simulink model "case8"  (R2024b)
settings: Solver=FixedStepAuto  StartTime=0  StopTime=1  FixedStep=1e-7  RelTol=1e-3
values from neighbouring files (symbols this model uses):
  SG_D_1_D = 0.01056    [IEEE9_case_parameters.m]    (also in case1_parameters.m; case2_parameters.m; case3_parameters.m; case4_parameters.m)
  SG_D_1_EnableSaturation = 0    [IEEE9_case_parameters.m]    (also in case1_parameters.m; case2_parameters.m; case3_parameters.m; case4_parameters.m)
  SG_D_1_f0 = 60    [IEEE9_case_parameters.m]    (also in case1_parameters.m; case2_parameters.m; case3_parameters.m; case4_parameters.m)
  SG_D_1_H = 7.5    [IEEE9_case_parameters.m]    (also in case1_parameters.m; case2_parameters.m; case3_parameters.m; case4_parameters.m)
  SG_D_1_K_A = 20    [IEEE9_case_parameters.m]    (also in case1_parameters.m; case2_parameters.m; case3_parameters.m; case4_parameters.m)
  SG_D_1_K_E = 1.000000e+1    (= 10)    [IEEE9_case_parameters.m]    (also in case1_parameters.m; case2_parameters.m; case3_parameters.m; case4_parameters.m)
  SG_D_1_K_F = 2.363    [IEEE9_case_parameters.m]    (also in case1_parameters.m; case2_parameters.m; case3_parameters.m; case4_parameters.m)
  SG_D_1_K_s = 0.5    [IEEE9_case_parameters.m]    (also in case1_parameters.m = 5; case2_parameters.m = 5; case3_parameters.m = 5; case4_parameters.m = 5)
  SG_D_1_R_a = 0.001088    [IEEE9_case_parameters.m]    (also in case1_parameters.m; case2_parameters.m; case3_parameters.m; case4_parameters.m)
  SG_D_1_S_A = 1    [IEEE9_case_parameters.m]    (also in case1_parameters.m; case2_parameters.m; case3_parameters.m; case4_parameters.m)
  SG_D_1_S_B = 0.103    [IEEE9_case_parameters.m]    (also in case1_parameters.m; case2_parameters.m; case3_parameters.m; case4_parameters.m)
  SG_D_1_S_N = 10.659857    [IEEE9_case_parameters.m]    (also in case1_parameters.m; case2_parameters.m; case3_parameters.m; case4_parameters.m)
  SG_D_1_SpeedPara = 200    [IEEE9_case_parameters.m]    (also in case1_parameters.m; case2_parameters.m; case3_parameters.m; case4_parameters.m)
  SG_D_1_T_0 = 0.720173    [IEEE9_case_parameters.m]    (also in case1_parameters.m = 0.755522; case2_parameters.m = 0.808931; case3_parameters.m = 0.869402; case4_parameters.m = 0.729316)
  SG_D_1_T_1 = 0.3    [IEEE9_case_parameters.m]    (also in case1_parameters.m; case2_parameters.m; case3_parameters.m; case4_parameters.m)
  SG_D_1_T_2 = 0.05    [IEEE9_case_parameters.m]    (also in case1_parameters.m; case2_parameters.m; case3_parameters.m; case4_parameters.m)
  SG_D_1_T_3 = 0.02    [IEEE9_case_parameters.m]    (also in case1_parameters.m; case2_parameters.m; case3_parameters.m; case4_parameters.m)
  SG_D_1_T_4 = 0.005    [IEEE9_case_parameters.m]    (also in case1_parameters.m; case2_parameters.m; case3_parameters.m; case4_parameters.m)
  SG_D_1_T_A = 0.02    [IEEE9_case_parameters.m]    (also in case1_parameters.m; case2_parameters.m; case3_parameters.m; case4_parameters.m)
  SG_D_1_T_dd = 8.000000e+0    (= 8)    [IEEE9_case_parameters.m]    (also in case1_parameters.m; case2_parameters.m; case3_parameters.m; case4_parameters.m)
  SG_D_1_T_ddd = 0.04    [IEEE9_case_parameters.m]    (also in case1_parameters.m; case2_parameters.m; case3_parameters.m; case4_parameters.m)
  SG_D_1_T_E = 0.314    [IEEE9_case_parameters.m]    (also in case1_parameters.m; case2_parameters.m; case3_parameters.m; case4_parameters.m)
  SG_D_1_T_F = 0.35    [IEEE9_case_parameters.m]    (also in case1_parameters.m; case2_parameters.m; case3_parameters.m; case4_parameters.m)
  SG_D_1_T_qd = 0.8    [IEEE9_case_parameters.m]    (also in case1_parameters.m; case2_parameters.m; case3_parameters.m; case4_parameters.m)
  SG_D_1_T_qdd = 0.02    [IEEE9_case_parameters.m]    (also in case1_parameters.m; case2_parameters.m; case3_parameters.m; case4_parameters.m)
  SG_D_1_T_speed = 0.1    [IEEE9_case_parameters.m]    (also in case1_parameters.m = 200; case2_parameters.m = 200; case3_parameters.m = 200; case4_parameters.m = 200)
  SG_D_1_T_w = 0.5    [IEEE9_case_parameters.m]    (also in case1_parameters.m; case2_parameters.m; case3_parameters.m; case4_parameters.m)
  SG_D_1_V_ref = 1.990276    [IEEE9_case_parameters.m]    (also in case1_parameters.m = 2.042296; case2_parameters.m = 2.051388; case3_parameters.m = 2.089584; case4_parameters.m = 2.01845)
  SG_D_1_w_ref = 376.991118    [IEEE9_case_parameters.m]    (also in case1_parameters.m; case2_parameters.m; case3_parameters.m; case4_parameters.m)
  SG_D_1_wb = 6.000000e+1    (= 60)    [IEEE9_case_parameters.m]    (also in case1_parameters.m; case2_parameters.m; case3_parameters.m; case4_parameters.m)
  SG_D_1_x_d = 1.9    [IEEE9_case_parameters.m]    (also in case1_parameters.m; case2_parameters.m; case3_parameters.m; case4_parameters.m)
  SG_D_1_x_dd = 0.302    [IEEE9_case_parameters.m]    (also in case1_parameters.m; case2_parameters.m; case3_parameters.m; case4_parameters.m)
  SG_D_1_x_ddd = 0.204    [IEEE9_case_parameters.m]    (also in case1_parameters.m; case2_parameters.m; case3_parameters.m; case4_parameters.m)
  SG_D_1_x_l = 0.05    [IEEE9_case_parameters.m]    (also in case1_parameters.m; case2_parameters.m; case3_parameters.m; case4_parameters.m)
  SG_D_1_x_q = 1.3    [IEEE9_case_parameters.m]    (also in case1_parameters.m; case2_parameters.m; case3_parameters.m; case4_parameters.m)
  SG_D_1_x_qd = 0.5    [IEEE9_case_parameters.m]    (also in case1_parameters.m; case2_parameters.m; case3_parameters.m; case4_parameters.m)
  SG_D_1_x_qdd = 0.3    [IEEE9_case_parameters.m]    (also in case1_parameters.m; case2_parameters.m; case3_parameters.m; case4_parameters.m)
  SG_D_2_D = 0.02    [IEEE9_case_parameters.m]    (also in case1_parameters.m; case2_parameters.m; case3_parameters.m; case4_parameters.m)
  SG_D_2_EnableSaturation = 0    [IEEE9_case_parameters.m]    (also in case1_parameters.m; case2_parameters.m; case3_parameters.m; case4_parameters.m)
  SG_D_2_f0 = 60    [IEEE9_case_parameters.m]    (also in case1_parameters.m; case2_parameters.m; case3_parameters.m; case4_parameters.m)
  SG_D_2_H = 8.000000e+0    (= 8)    [IEEE9_case_parameters.m]    (also in case1_parameters.m; case2_parameters.m; case3_parameters.m; case4_parameters.m)
  SG_D_2_K_A = 20    [IEEE9_case_parameters.m]    (also in case1_parameters.m; case2_parameters.m; case3_parameters.m; case4_parameters.m)
  SG_D_2_K_E = 1.000000e+1    (= 10)    [IEEE9_case_parameters.m]    (also in case1_parameters.m; case2_parameters.m; case3_parameters.m; case4_parameters.m)
  SG_D_2_K_F = 2.363    [IEEE9_case_parameters.m]    (also in case1_parameters.m; case2_parameters.m; case3_parameters.m; case4_parameters.m)
  SG_D_2_K_s = 0.5    [IEEE9_case_parameters.m]    (also in case1_parameters.m = 4; case2_parameters.m = 4; case3_parameters.m = 4; case4_parameters.m = 4)
  SG_D_2_R_a = 0.001088    [IEEE9_case_parameters.m]    (also in case1_parameters.m; case2_parameters.m; case3_parameters.m; case4_parameters.m)
  SG_D_2_S_A = 1    [IEEE9_case_parameters.m]    (also in case1_parameters.m; case2_parameters.m; case3_parameters.m; case4_parameters.m)
  SG_D_2_S_B = 0.103    [IEEE9_case_parameters.m]    (also in case1_parameters.m; case2_parameters.m; case3_parameters.m; case4_parameters.m)
  SG_D_2_S_N = 10.659857    [IEEE9_case_parameters.m]    (also in case1_parameters.m; case2_parameters.m; case3_parameters.m; case4_parameters.m)
  SG_D_2_SpeedPara = 200    [IEEE9_case_parameters.m]    (also in case1_parameters.m; case2_parameters.m; case3_parameters.m; case4_parameters.m)
  SG_D_2_T_0 = 1.632913    [IEEE9_case_parameters.m]    (also in case1_parameters.m = 1.632925; case2_parameters.m = 1.632915; case3_parameters.m = 1.632914; case4_parameters.m = 1.632927)
  SG_D_2_T_1 = 0.2    [IEEE9_case_parameters.m]    (also in case1_parameters.m; case2_parameters.m; case3_parameters.m; case4_parameters.m)
  SG_D_2_T_2 = 0.05    [IEEE9_case_parameters.m]    (also in case1_parameters.m; case2_parameters.m; case3_parameters.m; case4_parameters.m)
  SG_D_2_T_3 = 0.02    [IEEE9_case_parameters.m]    (also in case1_parameters.m; case2_parameters.m; case3_parameters.m; case4_parameters.m)
  SG_D_2_T_4 = 0.005    [IEEE9_case_parameters.m]    (also in case1_parameters.m; case2_parameters.m; case3_parameters.m; case4_parameters.m)
  SG_D_2_T_A = 0.02    [IEEE9_case_parameters.m]    (also in case1_parameters.m; case2_parameters.m; case3_parameters.m; case4_parameters.m)
  SG_D_2_T_dd = 7.9    [IEEE9_case_parameters.m]    (also in case1_parameters.m; case2_parameters.m; case3_parameters.m; case4_parameters.m)
  SG_D_2_T_ddd = 0.04    [IEEE9_case_parameters.m]    (also in case1_parameters.m; case2_parameters.m; case3_parameters.m; case4_parameters.m)
  SG_D_2_T_E = 0.314    [IEEE9_case_parameters.m]    (also in case1_parameters.m; case2_parameters.m; case3_parameters.m; case4_parameters.m)
  SG_D_2_T_F = 0.35    [IEEE9_case_parameters.m]    (also in case1_parameters.m; case2_parameters.m; case3_parameters.m; case4_parameters.m)
  SG_D_2_T_qd = 0.8    [IEEE9_case_parameters.m]    (also in case1_parameters.m; case2_parameters.m; case3_parameters.m; case4_parameters.m)
  SG_D_2_T_qdd = 0.015    [IEEE9_case_parameters.m]    (also in case1_parameters.m; case2_parameters.m; case3_parameters.m; case4_parameters.m)
  SG_D_2_T_speed = 0.1    [IEEE9_case_parameters.m]    (also in case1_parameters.m = 150; case2_parameters.m = 150; case3_parameters.m = 150; case4_parameters.m = 150)
  SG_D_2_T_w = 0.35    [IEEE9_case_parameters.m]    (also in case1_parameters.m; case2_parameters.m; case3_parameters.m; case4_parameters.m)
  SG_D_2_V_ref = 2.58547    [IEEE9_case_parameters.m]    (also in case1_parameters.m = 2.597896; case2_parameters.m = 2.587136; case3_parameters.m = 2.586042; case4_parameters.m = 2.599679)
  SG_D_2_w_ref = 376.991118    [IEEE9_case_parameters.m]    (also in case1_parameters.m; case2_parameters.m; case3_parameters.m; case4_parameters.m)
  SG_D_2_wb = 6.000000e+1    (= 60)    [IEEE9_case_parameters.m]    (also in case1_parameters.m; case2_parameters.m; case3_parameters.m; case4_parameters.m)
  SG_D_2_x_d = 1.8    [IEEE9_case_parameters.m]    (also in case1_parameters.m; case2_parameters.m; case3_parameters.m; case4_parameters.m)
  SG_D_2_x_dd = 0.302    [IEEE9_case_parameters.m]    (also in case1_parameters.m; case2_parameters.m; case3_parameters.m; case4_parameters.m)
  SG_D_2_x_ddd = 0.204    [IEEE9_case_parameters.m]    (also in case1_parameters.m; case2_parameters.m; case3_parameters.m; case4_parameters.m)
  SG_D_2_x_l = 0.05    [IEEE9_case_parameters.m]    (also in case1_parameters.m; case2_parameters.m; case3_parameters.m; case4_parameters.m)
  SG_D_2_x_q = 1.25    [IEEE9_case_parameters.m]    (also in case1_parameters.m; case2_parameters.m; case3_parameters.m; case4_parameters.m)
  SG_D_2_x_qd = 0.5    [IEEE9_case_parameters.m]    (also in case1_parameters.m; case2_parameters.m; case3_parameters.m; case4_parameters.m)
  SG_D_2_x_qdd = 0.3    [IEEE9_case_parameters.m]    (also in case1_parameters.m; case2_parameters.m; case3_parameters.m; case4_parameters.m)
  SG_D_3_D = 0.02    [IEEE9_case_parameters.m]    (also in case1_parameters.m; case2_parameters.m; case3_parameters.m; case4_parameters.m)
  SG_D_3_EnableSaturation = 0    [IEEE9_case_parameters.m]    (also in case1_parameters.m; case2_parameters.m; case3_parameters.m; case4_parameters.m)
  SG_D_3_f0 = 60    [IEEE9_case_parameters.m]    (also in case1_parameters.m; case2_parameters.m; case3_parameters.m; case4_parameters.m)
  SG_D_3_H = 7.7    [IEEE9_case_parameters.m]    (also in case1_parameters.m; case2_parameters.m; case3_parameters.m; case4_parameters.m)
  SG_D_3_K_A = 20    [IEEE9_case_parameters.m]    (also in case1_parameters.m; case2_parameters.m; case3_parameters.m; case4_parameters.m)
  SG_D_3_K_E = 1.000000e+1    (= 10)    [IEEE9_case_parameters.m]    (also in case1_parameters.m; case2_parameters.m; case3_parameters.m; case4_parameters.m)
  SG_D_3_K_F = 2.363    [IEEE9_case_parameters.m]    (also in case1_parameters.m; case2_parameters.m; case3_parameters.m; case4_parameters.m)
  SG_D_3_K_s = 0.2    [IEEE9_case_parameters.m]    (also in case1_parameters.m = 2; case2_parameters.m = 2; case3_parameters.m = 2; case4_parameters.m = 2)
  SG_D_3_R_a = 0.001088    [IEEE9_case_parameters.m]    (also in case1_parameters.m; case2_parameters.m; case3_parameters.m; case4_parameters.m)
  SG_D_3_S_A = 1    [IEEE9_case_parameters.m]    (also in case1_parameters.m; case2_parameters.m; case3_parameters.m; case4_parameters.m)
  SG_D_3_S_B = 0.103    [IEEE9_case_parameters.m]    (also in case1_parameters.m; case2_parameters.m; case3_parameters.m; case4_parameters.m)
  SG_D_3_S_N = 10.659857    [IEEE9_case_parameters.m]    (also in case1_parameters.m; case2_parameters.m; case3_parameters.m; case4_parameters.m)
  SG_D_3_SpeedPara = 200    [IEEE9_case_parameters.m]    (also in case1_parameters.m; case2_parameters.m; case3_parameters.m; case4_parameters.m)
  SG_D_3_T_0 = 0.850788    [IEEE9_case_parameters.m]    (also in case1_parameters.m = 0.850786; case2_parameters.m = 0.850787; case3_parameters.m; case4_parameters.m = 0.850786)
  SG_D_3_T_1 = 0.2    [IEEE9_case_parameters.m]    (also in case1_parameters.m; case2_parameters.m; case3_parameters.m; case4_parameters.m)
  SG_D_3_T_2 = 0.05    [IEEE9_case_parameters.m]    (also in case1_parameters.m; case2_parameters.m; case3_parameters.m; case4_parameters.m)
  SG_D_3_T_3 = 0.02    [IEEE9_case_parameters.m]    (also in case1_parameters.m; case2_parameters.m; case3_parameters.m; case4_parameters.m)
  SG_D_3_T_4 = 0.005    [IEEE9_case_parameters.m]    (also in case1_parameters.m; case2_parameters.m; case3_parameters.m; case4_parameters.m)
  SG_D_3_T_A = 0.02    [IEEE9_case_parameters.m]    (also in case1_parameters.m; case2_parameters.m; case3_parameters.m; case4_parameters.m)
  SG_D_3_T_dd = 8.1    [IEEE9_case_parameters.m]    (also in case1_parameters.m; case2_parameters.m; case3_parameters.m; case4_parameters.m)
  SG_D_3_T_ddd = 0.04    [IEEE9_case_parameters.m]    (also in case1_parameters.m; case2_parameters.m; case3_parameters.m; case4_parameters.m)
  SG_D_3_T_E = 0.314    [IEEE9_case_parameters.m]    (also in case1_parameters.m; case2_parameters.m; case3_parameters.m; case4_parameters.m)
  SG_D_3_T_F = 0.35    [IEEE9_case_parameters.m]    (also in case1_parameters.m; case2_parameters.m; case3_parameters.m; case4_parameters.m)
  SG_D_3_T_qd = 0.8    [IEEE9_case_parameters.m]    (also in case1_parameters.m; case2_parameters.m; case3_parameters.m; case4_parameters.m)
  SG_D_3_T_qdd = 0.015    [IEEE9_case_parameters.m]    (also in case1_parameters.m; case2_parameters.m; case3_parameters.m; case4_parameters.m)
  SG_D_3_T_speed = 0.1    [IEEE9_case_parameters.m]    (also in case1_parameters.m = 180; case2_parameters.m = 180; case3_parameters.m = 180; case4_parameters.m = 180)
  SG_D_3_T_w = 0.4    [IEEE9_case_parameters.m]    (also in case1_parameters.m; case2_parameters.m; case3_parameters.m; case4_parameters.m)
  SG_D_3_V_ref = 1.892727    [IEEE9_case_parameters.m]    (also in case1_parameters.m = 1.906439; case2_parameters.m = 1.895535; case3_parameters.m = 1.892105; case4_parameters.m = 1.906598)
  SG_D_3_w_ref = 376.991118    [IEEE9_case_parameters.m]    (also in case1_parameters.m; case2_parameters.m; case3_parameters.m; case4_parameters.m)
  SG_D_3_wb = 6.000000e+1    (= 60)    [IEEE9_case_parameters.m]    (also in case1_parameters.m; case2_parameters.m; case3_parameters.m; case4_parameters.m)
  SG_D_3_x_d = 1.85    [IEEE9_case_parameters.m]    (also in case1_parameters.m; case2_parameters.m; case3_parameters.m; case4_parameters.m)
  SG_D_3_x_dd = 0.302    [IEEE9_case_parameters.m]    (also in case1_parameters.m; case2_parameters.m; case3_parameters.m; case4_parameters.m)
  SG_D_3_x_ddd = 0.204    [IEEE9_case_parameters.m]    (also in case1_parameters.m; case2_parameters.m; case3_parameters.m; case4_parameters.m)
  SG_D_3_x_l = 0.05    [IEEE9_case_parameters.m]    (also in case1_parameters.m; case2_parameters.m; case3_parameters.m; case4_parameters.m)
  SG_D_3_x_q = 1.2    [IEEE9_case_parameters.m]    (also in case1_parameters.m; case2_parameters.m; case3_parameters.m; case4_parameters.m)
  SG_D_3_x_qd = 0.5    [IEEE9_case_parameters.m]    (also in case1_parameters.m; case2_parameters.m; case3_parameters.m; case4_parameters.m)
  SG_D_3_x_qdd = 0.3    [IEEE9_case_parameters.m]    (also in case1_parameters.m; case2_parameters.m; case3_parameters.m; case4_parameters.m)
(part 1 of 12)
settings Model: Creator=Greg  LastModifiedBy=Greg

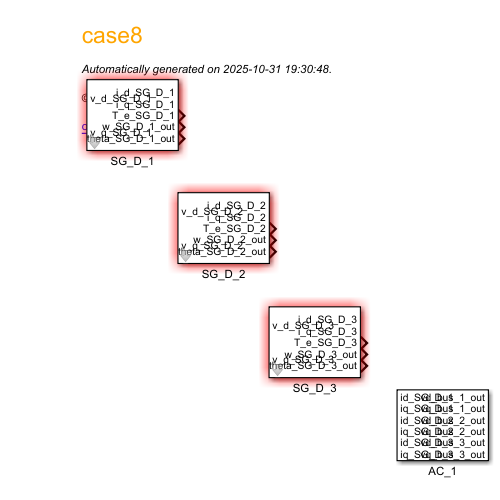
[thumbnail: Simulink's stored preview of the top-level diagram]
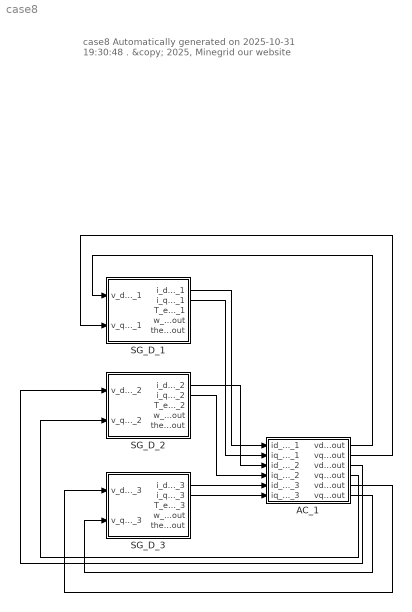
== system case8 ==
  note: case8
      | Automatically generated on 2025-10-31 19:30:48 .
      | &copy; 2025, Minegrid
      | our website
  AC_1 : Subsystem  mask(AC_1){}
      mask help: Parameters Interface of AC_1
  SG_D_1 : Subsystem  mask(SG_D_1){T_0=SG_D_1_T_0, w_ref=SG_D_1_w_ref, V_ref=SG_D_1_V_ref, x_d=SG_D_1_x_d, x_dd=SG_D_1_x_dd, x_ddd=SG_D_1_x_ddd, x_q=SG_D_1_x_q, x_qd=SG_D_1_x_qd, x_qdd=SG_D_1_x_qdd, x_l=SG_D_1_x_l, R_a=SG_D_1_R_a, T_dd=SG_D_1_T_dd, T_ddd=SG_D_1_T_ddd, T_qd=SG_D_1_T_qd, T_qdd=SG_D_1_T_qdd, H=SG_D_1_H, D=SG_D_1_D, SpeedPara=SG_D_1_SpeedPara, K_A=SG_D_1_K_A, EnableSaturation=SG_D_1_EnableSaturation, f0=SG_D_1_f0, T_speed=SG_D_1_T_speed, T_E=SG_D_1_T_E, T_A=SG_D_1_T_A, T_F=SG_D_1_T_F, K_E=SG_D_1_K_E, K_F=SG_D_1_K_F, K_s=SG_D_1_K_s, T_1=SG_D_1_T_1, T_2=SG_D_1_T_2, T_3=SG_D_1_T_3, T_4=SG_D_1_T_4, T_w=SG_D_1_T_w, wb=SG_D_1_wb, S_A=SG_D_1_S_A, S_B=SG_D_1_S_B, S_N=SG_D_1_S_N}
      mask help: Parameters Interface of SG_D_1
  SG_D_2 : Subsystem  mask(SG_D_2){T_0=SG_D_2_T_0, w_ref=SG_D_2_w_ref, V_ref=SG_D_2_V_ref, x_d=SG_D_2_x_d, x_dd=SG_D_2_x_dd, x_ddd=SG_D_2_x_ddd, x_q=SG_D_2_x_q, x_qd=SG_D_2_x_qd, x_qdd=SG_D_2_x_qdd, x_l=SG_D_2_x_l, R_a=SG_D_2_R_a, T_dd=SG_D_2_T_dd, T_ddd=SG_D_2_T_ddd, T_qd=SG_D_2_T_qd, T_qdd=SG_D_2_T_qdd, H=SG_D_2_H, D=SG_D_2_D, SpeedPara=SG_D_2_SpeedPara, K_A=SG_D_2_K_A, EnableSaturation=SG_D_2_EnableSaturation, f0=SG_D_2_f0, T_speed=SG_D_2_T_speed, T_E=SG_D_2_T_E, T_A=SG_D_2_T_A, T_F=SG_D_2_T_F, K_E=SG_D_2_K_E, K_F=SG_D_2_K_F, K_s=SG_D_2_K_s, T_1=SG_D_2_T_1, T_2=SG_D_2_T_2, T_3=SG_D_2_T_3, T_4=SG_D_2_T_4, T_w=SG_D_2_T_w, wb=SG_D_2_wb, S_A=SG_D_2_S_A, S_B=SG_D_2_S_B, S_N=SG_D_2_S_N}
      mask help: Parameters Interface of SG_D_2
  SG_D_3 : Subsystem  mask(SG_D_3){T_0=SG_D_3_T_0, w_ref=SG_D_3_w_ref, V_ref=SG_D_3_V_ref, x_d=SG_D_3_x_d, x_dd=SG_D_3_x_dd, x_ddd=SG_D_3_x_ddd, x_q=SG_D_3_x_q, x_qd=SG_D_3_x_qd, x_qdd=SG_D_3_x_qdd, x_l=SG_D_3_x_l, R_a=SG_D_3_R_a, T_dd=SG_D_3_T_dd, T_ddd=SG_D_3_T_ddd, T_qd=SG_D_3_T_qd, T_qdd=SG_D_3_T_qdd, H=SG_D_3_H, D=SG_D_3_D, SpeedPara=SG_D_3_SpeedPara, K_A=SG_D_3_K_A, EnableSaturation=SG_D_3_EnableSaturation, f0=SG_D_3_f0, T_speed=SG_D_3_T_speed, T_E=SG_D_3_T_E, T_A=SG_D_3_T_A, T_F=SG_D_3_T_F, K_E=SG_D_3_K_E, K_F=SG_D_3_K_F, K_s=SG_D_3_K_s, T_1=SG_D_3_T_1, T_2=SG_D_3_T_2, T_3=SG_D_3_T_3, T_4=SG_D_3_T_4, T_w=SG_D_3_T_w, wb=SG_D_3_wb, S_A=SG_D_3_S_A, S_B=SG_D_3_S_B, S_N=SG_D_3_S_N}
      mask help: Parameters Interface of SG_D_3
  wires:
  SG_D_2/2(i_q_SG_D_2) -> AC_1/4(iq_SG_D_2)
  SG_D_1/2(i_q_SG_D_1) -> AC_1/2(iq_SG_D_1)
  SG_D_1/1(i_d_SG_D_1) -> AC_1/1(id_SG_D_1)
  SG_D_2/1(i_d_SG_D_2) -> AC_1/3(id_SG_D_2)
  AC_1/1(vd_bus_1_out) -> SG_D_1/1(v_d_SG_D_1)
  SG_D_3/1(i_d_SG_D_3) -> AC_1/5(id_SG_D_3)
  AC_1/2(vq_bus_1_out) -> SG_D_1/2(v_q_SG_D_1)
  SG_D_3/2(i_q_SG_D_3) -> AC_1/6(iq_SG_D_3)
  AC_1/3(vd_bus_2_out) -> SG_D_2/1(v_d_SG_D_2)
  AC_1/4(vq_bus_2_out) -> SG_D_2/2(v_q_SG_D_2)
  AC_1/5(vd_bus_3_out) -> SG_D_3/1(v_d_SG_D_3)
  AC_1/6(vq_bus_3_out) -> SG_D_3/2(v_q_SG_D_3)

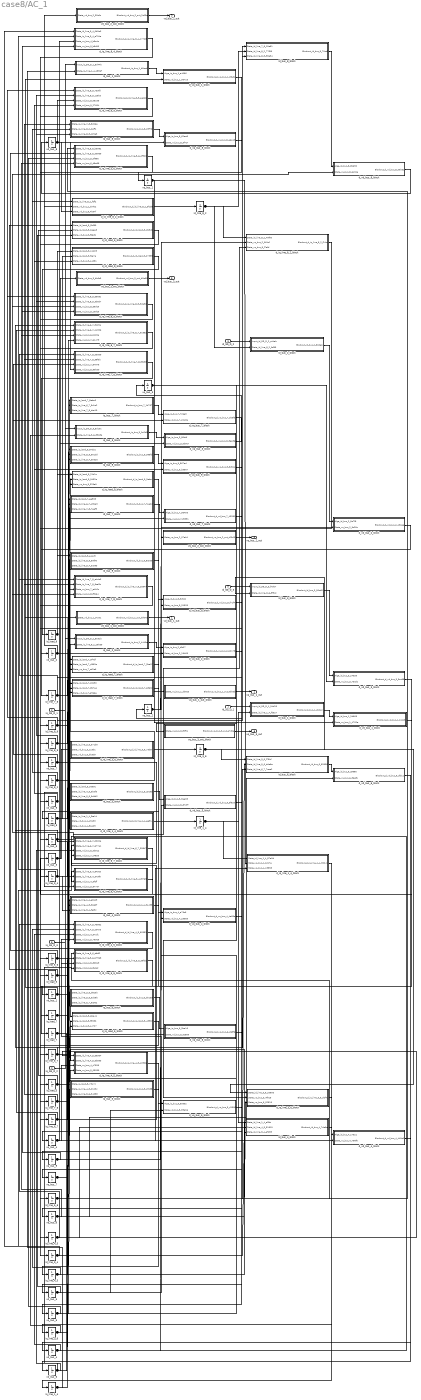
== system case8/AC_1 ==
  id_SG_D_1 : Inport
  iq_SG_D_1 : Inport  Port=2
  id_SG_D_2 : Inport  Port=3
  iq_SG_D_2 : Inport  Port=4
  id_SG_D_3 : Inport  Port=5
  iq_SG_D_3 : Inport  Port=6
  d_id_line_1_4_block : Subsystem
  d_id_line_3_6_block : Subsystem
  d_id_line_4_5_block : Subsystem
  d_id_line_5_6_block : Subsystem
  d_id_line_6_7_block : Subsystem
  d_id_line_7_8_block : Subsystem
  d_id_line_8_2_block : Subsystem
  d_id_line_8_9_block : Subsystem
  d_id_line_9_4_block : Subsystem
  d_id_load_5_block : Subsystem
  d_id_load_7_block : Subsystem
  d_id_load_9_block : Subsystem
  d_iq_line_1_4_block : Subsystem
  d_iq_line_3_6_block : Subsystem
  d_iq_line_4_5_block : Subsystem
  d_iq_line_5_6_block : Subsystem
  d_iq_line_6_7_block : Subsystem
  d_iq_line_7_8_block : Subsystem
  d_iq_line_8_2_block : Subsystem
  d_iq_line_8_9_block : Subsystem
  d_iq_line_9_4_block : Subsystem
  d_iq_load_5_block : Subsystem
  d_iq_load_7_block : Subsystem
  d_iq_load_9_block : Subsystem
  d_vd_bus_1_block : Subsystem
  d_vd_bus_2_block : Subsystem
  d_vd_bus_3_block : Subsystem
  d_vd_bus_4_block : Subsystem
  d_vd_bus_5_block : Subsystem
  d_vd_bus_6_block : Subsystem
  d_vd_bus_7_block : Subsystem
  d_vd_bus_8_block : Subsystem
  d_vd_bus_9_block : Subsystem
  d_vq_bus_1_block : Subsystem
  d_vq_bus_2_block : Subsystem
  d_vq_bus_3_block : Subsystem
  d_vq_bus_4_block : Subsystem
  d_vq_bus_5_block : Subsystem
  d_vq_bus_6_block : Subsystem
  d_vq_bus_7_block : Subsystem
  d_vq_bus_8_block : Subsystem
  d_vq_bus_9_block : Subsystem
  id_bus_1_block : Subsystem
  id_bus_2_block : Subsystem
  id_bus_3_block : Subsystem
  id_bus_4_block : Subsystem
  id_bus_5_block : Subsystem
  id_bus_6_block : Subsystem
  id_bus_7_block : Subsystem
  id_bus_8_block : Subsystem
  id_bus_9_block : Subsystem
  id_line_1_4 : Integrator  InitialCondition=0.683
  id_line_3_6 : Integrator  InitialCondition=0.8406
  id_line_4_5 : Integrator  InitialCondition=0.2917
  id_line_5_6 : Integrator  InitialCondition=-0.6125
  id_line_6_7 : Integrator  InitialCondition=0.2391
  id_line_7_8 : Integrator  InitialCondition=-0.763
  id_line_8_2 : Integrator  InitialCondition=-1.6242
  id_line_8_9 : Integrator  InitialCondition=0.8774
  id_line_9_4 : Integrator  InitialCondition=-0.3847
  id_load_5 : Integrator  InitialCondition=0.8871467636805124
  id_load_7 : Integrator  InitialCondition=1.0049034785630728
  id_load_9 : Integrator  InitialCondition=1.2451541471351033
  iq_bus_1_block : Subsystem
  iq_bus_2_block : Subsystem
  iq_bus_3_block : Subsystem
  iq_bus_4_block : Subsystem
  iq_bus_5_block : Subsystem
  iq_bus_6_block : Subsystem
  iq_bus_7_block : Subsystem
  iq_bus_8_block : Subsystem
  iq_bus_9_block : Subsystem
  iq_line_1_4 : Integrator  InitialCondition=-0.1786
  iq_line_3_6 : Integrator  InitialCondition=0.1439
  iq_line_4_5 : Integrator  InitialCondition=-0.064
  iq_line_5_6 : Integrator  InitialCondition=0.0192
  iq_line_6_7 : Integrator  InitialCondition=-0.1218
  iq_line_7_8 : Integrator  InitialCondition=0.0037
  iq_line_8_2 : Integrator  InitialCondition=-0.1756
  iq_line_8_9 : Integrator  InitialCondition=-0.0473
  iq_line_9_4 : Integrator  InitialCondition=0.2799
  iq_load_5 : Integrator  InitialCondition=-0.33570557583772886
  iq_load_7 : Integrator  InitialCondition=-0.30253966294593626
  iq_load_9 : Integrator  InitialCondition=-0.559052312749489
  vd_bus_1 : Integrator  InitialCondition=1.0
  vd_bus_1_out_block : Subsystem
  vd_bus_2 : Integrator  InitialCondition=0.9847356420938818
  vd_bus_2_out_block : Subsystem
  vd_bus_3 : Integrator  InitialCondition=0.9960672142876663
  vd_bus_3_out_block : Subsystem
  vd_bus_4 : Integrator  InitialCondition=0.9895844597843511
  vd_bus_5 : Integrator  InitialCondition=0.9789947177747443
  vd_bus_6 : Integrator  InitialCondition=1.0046035882492705
  vd_bus_7 : Integrator  InitialCondition=0.9895204593849437
  vd_bus_8 : Integrator  InitialCondition=0.9958449354757835
  vd_bus_9 : Integrator  InitialCondition=0.9619042233859942
  vq_bus_1 : Integrator  InitialCondition=0.0
  vq_bus_1_out_block : Subsystem
  vq_bus_2 : Integrator  InitialCondition=0.17405664362485687
  vq_bus_2_out_block : Subsystem
  vq_bus_3 : Integrator  InitialCondition=0.08860081614301404
  vq_bus_3_out_block : Subsystem
  vq_bus_4 : Integrator  InitialCondition=-0.0398310299723944
  vq_bus_5 : Integrator  InitialCondition=-0.06598398942448998
  vq_bus_6 : Integrator  InitialCondition=0.03873258011920573
  vq_bus_7 : Integrator  InitialCondition=0.01568979914580082
  vq_bus_8 : Integrator  InitialCondition=0.07128160735371208
  vq_bus_9 : Integrator  InitialCondition=-0.07032110002516861
  vd_bus_1_out : Outport
  vq_bus_1_out : Outport  Port=2
  vd_bus_2_out : Outport  Port=3
  vq_bus_2_out : Outport  Port=4
  vd_bus_3_out : Outport  Port=5
  vq_bus_3_out : Outport  Port=6
  wires:
  iq_bus_5_block/1(Blockout_iq_bus_5_2f438) -> d_vq_bus_5_block/1(Alge_iq_bus_5_593e2)
  d_id_line_1_4_block/1(Blockout_d_id_line_1_4_ee914) -> id_line_1_4/1
  vq_bus_2_out_block/1(Blockout_vq_bus_2_out_c20d3) -> vq_bus_2_out/1
  iq_SG_D_3/1 -> iq_bus_3_block/1(Input_iq_SG_D_3_5d10c)
  id_line_3_6/1 -> id_bus_3_block/2(State_id_line_3_6_5f9cc), id_bus_6_block/1(State_id_line_3_6_f75bf), d_iq_line_3_6_block/1(State_id_line_3_6_2080e)
  vd_bus_3_out_block/1(Blockout_vd_bus_3_out_b3a99) -> vd_bus_3_out/1
  d_iq_line_8_2_block/1(Blockout_d_iq_line_8_2_f14cf) -> iq_line_8_2/1
  d_vd_bus_4_block/1(Blockout_d_vd_bus_4_449c0) -> vd_bus_4/1
  id_SG_D_3/1 -> id_bus_3_block/1(Input_id_SG_D_3_f75b7)
  id_load_5/1 -> d_id_load_5_block/1(State_id_load_5_5bf89), d_iq_load_5_block/1(State_id_load_5_6ba41), id_bus_5_block/1(State_id_load_5_a095c)
  iq_bus_3_block/1(Blockout_iq_bus_3_1a2d8) -> d_vq_bus_3_block/1(Alge_iq_bus_3_80dcf)
  d_id_load_7_block/1(Blockout_d_id_load_7_6563c) -> id_load_7/1
  iq_bus_6_block/1(Blockout_iq_bus_6_da1e9) -> d_vq_bus_6_block/1(Alge_iq_bus_6_3ba16)
  id_line_8_9/1 -> d_id_line_8_9_block/1(State_id_line_8_9_733fd), d_iq_line_8_9_block/1(State_id_line_8_9_e905c), id_bus_9_block/2(State_id_line_8_9_50f90), id_bus_8_block/3(State_id_line_8_9_98e94)
  id_line_9_4/1 -> d_id_line_9_4_block/1(State_id_line_9_4_843c0), d_iq_line_9_4_block/1(State_id_line_9_4_0b3a3), id_bus_4_block/3(State_id_line_9_4_afd85), id_bus_9_block/3(State_id_line_9_4_ac093)
  vq_bus_8/1 -> d_vd_bus_8_block/2(State_vq_bus_8_643ce), d_iq_line_7_8_block/4(State_vq_bus_8_f3b64), d_iq_line_8_9_block/3(State_vq_bus_8_e6dc9), d_iq_line_8_2_block/3(State_vq_bus_8_f7efd)
  iq_SG_D_2/1 -> iq_bus_2_block/1(Input_iq_SG_D_2_5a31b)
  id_line_6_7/1 -> d_id_line_6_7_block/1(State_id_line_6_7_0b02a), d_iq_line_6_7_block/1(State_id_line_6_7_9c15a), id_bus_7_block/2(State_id_line_6_7_45ba3), id_bus_6_block/3(State_id_line_6_7_7cee2)
  id_bus_2_block/1(Blockout_id_bus_2_80de6) -> d_vd_bus_2_block/1(Alge_id_bus_2_5a7f8)
  iq_bus_4_block/1(Blockout_iq_bus_4_34493) -> d_vq_bus_4_block/1(Alge_iq_bus_4_a79c6)
  id_bus_9_block/1(Blockout_id_bus_9_8caa0) -> d_vd_bus_9_block/1(Alge_id_bus_9_9c9c2)
  iq_SG_D_1/1 -> iq_bus_1_block/1(Input_iq_SG_D_1_5d44b)
  d_id_line_4_5_block/1(Blockout_d_id_line_4_5_60351) -> id_line_4_5/1
  id_SG_D_2/1 -> id_bus_2_block/1(Input_id_SG_D_2_c44ab)
  id_SG_D_1/1 -> id_bus_1_block/1(Input_id_SG_D_1_34d26)
  id_load_9/1 -> d_id_load_9_block/1(State_id_load_9_11d25), id_bus_9_block/1(State_id_load_9_a44c9), d_iq_load_9_block/1(State_id_load_9_21d1c)
  vd_bus_1_out_block/1(Blockout_vd_bus_1_out_dd07e) -> vd_bus_1_out/1
  id_bus_4_block/1(Blockout_id_bus_4_7de9e) -> d_vd_bus_4_block/1(Alge_id_bus_4_17e21)
  vq_bus_1_out_block/1(Blockout_vq_bus_1_out_0bb6b) -> vq_bus_1_out/1
  d_iq_line_1_4_block/1(Blockout_d_iq_line_1_4_90247) -> iq_line_1_4/1
  id_line_4_5/1 -> d_id_line_4_5_block/1(State_id_line_4_5_4e862), d_iq_line_4_5_block/1(State_id_line_4_5_e9364), id_bus_4_block/2(State_id_line_4_5_51819), id_bus_5_block/2(State_id_line_4_5_ebaf3)
  id_bus_6_block/1(Blockout_id_bus_6_83936) -> d_vd_bus_6_block/1(Alge_id_bus_6_c988e)
  d_id_load_9_block/1(Blockout_d_id_load_9_27399) -> id_load_9/1
  vd_bus_7/1 -> d_vq_bus_7_block/2(State_vd_bus_7_2248a), d_id_line_7_8_block/3(State_vd_bus_7_87876), d_id_load_7_block/3(State_vd_bus_7_a966e), d_id_line_6_7_block/4(State_vd_bus_7_c4833)
  iq_bus_9_block/1(Blockout_iq_bus_9_995fd) -> d_vq_bus_9_block/1(Alge_iq_bus_9_567ad)
  vq_bus_3_out_block/1(Blockout_vq_bus_3_out_a7c8e) -> vq_bus_3_out/1
  iq_bus_8_block/1(Blockout_iq_bus_8_09f70) -> d_vq_bus_8_block/1(Alge_iq_bus_8_62ae5)
  iq_line_5_6/1 -> d_id_line_5_6_block/2(State_iq_line_5_6_b7968), d_iq_line_5_6_block/2(State_iq_line_5_6_a09e9), iq_bus_5_block/3(State_iq_line_5_6_34d88), iq_bus_6_block/2(State_iq_line_5_6_a2b8b)
  id_bus_3_block/1(Blockout_id_bus_3_50cd8) -> d_vd_bus_3_block/1(Alge_id_bus_3_24e35)
  id_bus_8_block/1(Blockout_id_bus_8_70ccf) -> d_vd_bus_8_block/1(Alge_id_bus_8_8b650)
  iq_line_9_4/1 -> d_id_line_9_4_block/2(State_iq_line_9_4_373f8), d_iq_line_9_4_block/2(State_iq_line_9_4_e794a), iq_bus_4_block/3(State_iq_line_9_4_fec9c), iq_bus_9_block/3(State_iq_line_9_4_3ae2e)
  d_iq_line_3_6_block/1(Blockout_d_iq_line_3_6_dcf40) -> iq_line_3_6/1
  vq_bus_6/1 -> d_iq_line_3_6_block/3(State_vq_bus_6_02815), d_vd_bus_6_block/2(State_vq_bus_6_96ef6), d_iq_line_5_6_block/4(State_vq_bus_6_d8e58), d_iq_line_6_7_block/3(State_vq_bus_6_bc18e)
  iq_bus_7_block/1(Blockout_iq_bus_7_1d767) -> d_vq_bus_7_block/1(Alge_iq_bus_7_726e3)
  iq_load_7/1 -> d_iq_load_7_block/2(State_iq_load_7_d963a), iq_bus_7_block/1(State_iq_load_7_8eba6), d_id_load_7_block/2(State_iq_load_7_8b7e4)
  id_bus_7_block/1(Blockout_id_bus_7_7ae2c) -> d_vd_bus_7_block/1(Alge_id_bus_7_9e4a6)
  id_bus_5_block/1(Blockout_id_bus_5_cac9d) -> d_vd_bus_5_block/1(Alge_id_bus_5_9ae33)
  id_line_7_8/1 -> id_bus_8_block/1(State_id_line_7_8_15e81), d_id_line_7_8_block/1(State_id_line_7_8_aae09), id_bus_7_block/3(State_id_line_7_8_7eef9), d_iq_line_7_8_block/1(State_id_line_7_8_e4da3)
  iq_bus_2_block/1(Blockout_iq_bus_2_4440e) -> d_vq_bus_2_block/1(Alge_iq_bus_2_dfc07)
  iq_line_6_7/1 -> d_id_line_6_7_block/2(State_iq_line_6_7_677a1), iq_bus_6_block/3(State_iq_line_6_7_6c502), iq_bus_7_block/2(State_iq_line_6_7_5c1a2), d_iq_line_6_7_block/2(State_iq_line_6_7_14306)
  d_iq_line_7_8_block/1(Blockout_d_iq_line_7_8_2e847) -> iq_line_7_8/1
  vd_bus_2_out_block/1(Blockout_vd_bus_2_out_2c03e) -> vd_bus_2_out/1
  iq_line_8_2/1 -> d_id_line_8_2_block/1(State_iq_line_8_2_fcff2), iq_bus_8_block/2(State_iq_line_8_2_2aff1), iq_bus_2_block/2(State_iq_line_8_2_29be9)
  iq_bus_1_block/1(Blockout_iq_bus_1_b5acd) -> d_vq_bus_1_block/1(Alge_iq_bus_1_a4066)
  d_iq_load_9_block/1(Blockout_d_iq_load_9_3eba4) -> iq_load_9/1
  iq_line_7_8/1 -> d_id_line_7_8_block/2(State_iq_line_7_8_58fab), d_iq_line_7_8_block/2(State_iq_line_7_8_8ce3b), iq_bus_7_block/3(State_iq_line_7_8_dca19), iq_bus_8_block/1(State_iq_line_7_8_8d26a)
  id_bus_1_block/1(Blockout_id_bus_1_cb042) -> d_vd_bus_1_block/1(Alge_id_bus_1_2d668)
  iq_line_1_4/1 -> d_id_line_1_4_block/1(State_iq_line_1_4_fbe14), iq_bus_1_block/2(State_iq_line_1_4_1856f), iq_bus_4_block/1(State_iq_line_1_4_e84c9)
  d_id_line_8_2_block/1(Blockout_d_id_line_8_2_3fcd8) -> id_line_8_2/1
  d_id_line_3_6_block/1(Blockout_d_id_line_3_6_73b84) -> id_line_3_6/1
  vq_bus_3/1 -> d_vd_bus_3_block/2(State_vq_bus_3_73cd2), vq_bus_3_out_block/1(State_vq_bus_3_f0f91), d_iq_line_3_6_block/2(State_vq_bus_3_4f015)
  iq_line_8_9/1 -> d_iq_line_8_9_block/2(State_iq_line_8_9_3bed7), iq_bus_8_block/3(State_iq_line_8_9_c19e3), iq_bus_9_block/2(State_iq_line_8_9_901dd), d_id_line_8_9_block/2(State_iq_line_8_9_1c9ba)
  vd_bus_1/1 -> d_vq_bus_1_block/2(State_vd_bus_1_06716), d_id_line_1_4_block/2(State_vd_bus_1_49433), vd_bus_1_out_block/1(State_vd_bus_1_c7201)
  vd_bus_4/1 -> d_id_line_1_4_block/3(State_vd_bus_4_56409), d_id_line_4_5_block/3(State_vd_bus_4_571f1), d_id_line_9_4_block/3(State_vd_bus_4_5fcff), d_vq_bus_4_block/2(State_vd_bus_4_25e83)
  id_line_8_2/1 -> d_iq_line_8_2_block/1(State_id_line_8_2_40f60), id_bus_2_block/2(State_id_line_8_2_faf95), id_bus_8_block/2(State_id_line_8_2_77f88)
  vq_bus_9/1 -> d_vd_bus_9_block/2(State_vq_bus_9_31533), d_iq_load_9_block/3(State_vq_bus_9_325e9), d_iq_line_9_4_block/4(State_vq_bus_9_b8c36), d_iq_line_8_9_block/4(State_vq_bus_9_10dc5)
  iq_line_3_6/1 -> d_id_line_3_6_block/1(State_iq_line_3_6_a71b0), iq_bus_3_block/2(State_iq_line_3_6_5365a), iq_bus_6_block/1(State_iq_line_3_6_d82ab)
  id_line_5_6/1 -> id_bus_6_block/2(State_id_line_5_6_dde6e), d_id_line_5_6_block/1(State_id_line_5_6_cfe92), d_iq_line_5_6_block/1(State_id_line_5_6_be082), id_bus_5_block/3(State_id_line_5_6_9ddb2)
  iq_line_4_5/1 -> d_id_line_4_5_block/2(State_iq_line_4_5_c67ae), d_iq_line_4_5_block/2(State_iq_line_4_5_eb553), iq_bus_4_block/2(State_iq_line_4_5_3660f), iq_bus_5_block/2(State_iq_line_4_5_0123c)
  d_id_line_9_4_block/1(Blockout_d_id_line_9_4_fd769) -> id_line_9_4/1
  vq_bus_5/1 -> d_vd_bus_5_block/2(State_vq_bus_5_87df7), d_iq_load_5_block/3(State_vq_bus_5_44727), d_iq_line_4_5_block/4(State_vq_bus_5_05939), d_iq_line_5_6_block/3(State_vq_bus_5_af966)
  id_line_1_4/1 -> d_iq_line_1_4_block/1(State_id_line_1_4_87a5d), id_bus_1_block/2(State_id_line_1_4_fde27), id_bus_4_block/1(State_id_line_1_4_affcb)
  vd_bus_6/1 -> d_vq_bus_6_block/2(State_vd_bus_6_0c589), d_id_line_3_6_block/3(State_vd_bus_6_bb3d9), d_id_line_6_7_block/3(State_vd_bus_6_ab512), d_id_line_5_6_block/4(State_vd_bus_6_fecad)
  iq_load_9/1 -> d_id_load_9_block/2(State_iq_load_9_fce7e), d_iq_load_9_block/2(State_iq_load_9_9492a), iq_bus_9_block/1(State_iq_load_9_87d2c)
  id_load_7/1 -> d_id_load_7_block/1(State_id_load_7_02c90), d_iq_load_7_block/1(State_id_load_7_0f4df), id_bus_7_block/1(State_id_load_7_ee538)
  iq_load_5/1 -> d_id_load_5_block/2(State_iq_load_5_baea8), d_iq_load_5_block/2(State_iq_load_5_f938b), iq_bus_5_block/1(State_iq_load_5_7347c)
  vd_bus_5/1 -> d_vq_bus_5_block/2(State_vd_bus_5_59ab6), d_id_load_5_block/3(State_vd_bus_5_fd6db), d_id_line_4_5_block/4(State_vd_bus_5_769c8), d_id_line_5_6_block/3(State_vd_bus_5_80849)
  vd_bus_9/1 -> d_vq_bus_9_block/2(State_vd_bus_9_b5567), d_id_load_9_block/3(State_vd_bus_9_44d81), d_id_line_8_9_block/4(State_vd_bus_9_27604), d_id_line_9_4_block/4(State_vd_bus_9_877a7)
  vd_bus_2/1 -> d_vq_bus_2_block/2(State_vd_bus_2_19465), vd_bus_2_out_block/1(State_vd_bus_2_35c0c), d_id_line_8_2_block/2(State_vd_bus_2_dc4b2)
  vd_bus_8/1 -> d_vq_bus_8_block/2(State_vd_bus_8_5f7c7), d_id_line_7_8_block/4(State_vd_bus_8_80ba0), d_id_line_8_2_block/3(State_vd_bus_8_4b57f), d_id_line_8_9_block/3(State_vd_bus_8_052a5)
  vq_bus_7/1 -> d_vd_bus_7_block/2(State_vq_bus_7_fd391), d_iq_load_7_block/3(State_vq_bus_7_cd2e6), d_iq_line_6_7_block/4(State_vq_bus_7_61479), d_iq_line_7_8_block/3(State_vq_bus_7_e4b2c)
  vq_bus_4/1 -> d_vd_bus_4_block/2(State_vq_bus_4_796f6), d_iq_line_1_4_block/3(State_vq_bus_4_19898), d_iq_line_4_5_block/3(State_vq_bus_4_c7938), d_iq_line_9_4_block/3(State_vq_bus_4_b5a4c)
  vd_bus_3/1 -> d_vq_bus_3_block/2(State_vd_bus_3_0b9c7), d_id_line_3_6_block/2(State_vd_bus_3_123b1), vd_bus_3_out_block/1(State_vd_bus_3_bb6c5)
  vq_bus_2/1 -> d_vd_bus_2_block/2(State_vq_bus_2_9c28c), d_iq_line_8_2_block/2(State_vq_bus_2_064cf), vq_bus_2_out_block/1(State_vq_bus_2_07eb1)
  vq_bus_1/1 -> d_iq_line_1_4_block/2(State_vq_bus_1_bc17e), d_vd_bus_1_block/2(State_vq_bus_1_4702e), vq_bus_1_out_block/1(State_vq_bus_1_dbece)
  d_iq_line_9_4_block/1(Blockout_d_iq_line_9_4_17728) -> iq_line_9_4/1
  d_vq_bus_7_block/1(Blockout_d_vq_bus_7_abefa) -> vq_bus_7/1
  d_vq_bus_2_block/1(Blockout_d_vq_bus_2_b2178) -> vq_bus_2/1
  d_iq_line_5_6_block/1(Blockout_d_iq_line_5_6_2f920) -> iq_line_5_6/1
  d_vq_bus_4_block/1(Blockout_d_vq_bus_4_4e85a) -> vq_bus_4/1
  d_iq_line_8_9_block/1(Blockout_d_iq_line_8_9_9da92) -> iq_line_8_9/1
  d_iq_load_5_block/1(Blockout_d_iq_load_5_439b9) -> iq_load_5/1
  d_id_line_5_6_block/1(Blockout_d_id_line_5_6_a6fd1) -> id_line_5_6/1
  d_id_line_6_7_block/1(Blockout_d_id_line_6_7_39847) -> id_line_6_7/1
  d_id_load_5_block/1(Blockout_d_id_load_5_0b5cb) -> id_load_5/1
  d_id_line_8_9_block/1(Blockout_d_id_line_8_9_aecdd) -> id_line_8_9/1
  d_vd_bus_3_block/1(Blockout_d_vd_bus_3_5ac98) -> vd_bus_3/1
  d_iq_line_6_7_block/1(Blockout_d_iq_line_6_7_91852) -> iq_line_6_7/1
  d_id_line_7_8_block/1(Blockout_d_id_line_7_8_fdb38) -> id_line_7_8/1
  d_iq_line_4_5_block/1(Blockout_d_iq_line_4_5_40906) -> iq_line_4_5/1
  d_iq_load_7_block/1(Blockout_d_iq_load_7_3ba97) -> iq_load_7/1
  d_vq_bus_6_block/1(Blockout_d_vq_bus_6_d63f6) -> vq_bus_6/1
  d_vd_bus_5_block/1(Blockout_d_vd_bus_5_3f620) -> vd_bus_5/1
  d_vq_bus_3_block/1(Blockout_d_vq_bus_3_9ea56) -> vq_bus_3/1
  d_vd_bus_2_block/1(Blockout_d_vd_bus_2_136aa) -> vd_bus_2/1
  d_vd_bus_1_block/1(Blockout_d_vd_bus_1_b1cc3) -> vd_bus_1/1
  d_vd_bus_6_block/1(Blockout_d_vd_bus_6_cfd11) -> vd_bus_6/1
  d_vq_bus_9_block/1(Blockout_d_vq_bus_9_8c5c4) -> vq_bus_9/1
  d_vd_bus_7_block/1(Blockout_d_vd_bus_7_43381) -> vd_bus_7/1
  d_vd_bus_8_block/1(Blockout_d_vd_bus_8_aabe1) -> vd_bus_8/1
  d_vd_bus_9_block/1(Blockout_d_vd_bus_9_f71f4) -> vd_bus_9/1
  d_vq_bus_1_block/1(Blockout_d_vq_bus_1_0fecb) -> vq_bus_1/1
  d_vq_bus_5_block/1(Blockout_d_vq_bus_5_d199f) -> vq_bus_5/1
  d_vq_bus_8_block/1(Blockout_d_vq_bus_8_a6a13) -> vq_bus_8/1

== system case8/SG_D_1 ==
  v_d_SG_D_1 : Inport
  v_q_SG_D_1 : Inport  Port=2
  E_fd_SG_D_1 : Integrator  InitialCondition=1.8457126523459264
  Px_1_SG_D_1 : Integrator  InitialCondition=0.0
  Px_2_SG_D_1 : Integrator  InitialCondition=0.0
  Px_3_SG_D_1 : Integrator  InitialCondition=5.162338753620879e-26
  R_f_SG_D_1 : Integrator  InitialCondition=12.4611971356955
  T_e_SG_D_1_block : Subsystem
  T_m_SG_D_1 : Integrator  InitialCondition=0.6835726709725602
  V_f_SG_D_1 : Integrator  InitialCondition=18.457126523459266
  d_E_fd_SG_D_1_block : Subsystem
  d_Px_1_SG_D_1_block : Subsystem
  d_Px_2_SG_D_1_block : Subsystem
  d_Px_3_SG_D_1_block : Subsystem
  d_R_f_SG_D_1_block : Subsystem
  d_T_m_SG_D_1_block : Subsystem
  d_V_f_SG_D_1_block : Subsystem
  d_psi_1d_SG_D_1_block : Subsystem
  d_psi_d_SG_D_1_block : Subsystem
  d_psi_fd_SG_D_1_block : Subsystem
  d_psi_gq_SG_D_1_block : Subsystem
  d_psi_kq_SG_D_1_block : Subsystem
  d_psi_q_SG_D_1_block : Subsystem
  d_theta_SG_D_1_block : Subsystem
  d_w_SG_D_1_block : Subsystem
  i_d_SG_D_1_block : Subsystem
  i_q_SG_D_1_block : Subsystem
  psi_1d_SG_D_1 : Integrator  InitialCondition=0.8392160975173428
  psi_d_SG_D_1 : Integrator  InitialCondition=0.8120134879273809
  psi_fd_SG_D_1 : Integrator  InitialCondition=0.97631724985075
  psi_gq_SG_D_1 : Integrator  InitialCondition=0.359945273705796
  psi_kq_SG_D_1 : Integrator  InitialCondition=-0.5624144901653062
  psi_q_SG_D_1 : Integrator  InitialCondition=-0.5849110697719185
  theta_SG_D_1 : Integrator  InitialCondition=0.6240408159147169
  theta_SG_D_1_out_block : Subsystem
  w_SG_D_1 : Integrator  InitialCondition=376.99111843077515
  w_SG_D_1_out_block : Subsystem
  i_d_SG_D_1 : Outport
  i_q_SG_D_1 : Outport  Port=2
  T_e_SG_D_1 : Outport  Port=3
  w_SG_D_1_out : Outport  Port=4
  theta_SG_D_1_out : Outport  Port=5
  wires:
  V_f_SG_D_1/1 -> d_V_f_SG_D_1_block/14(State_V_f_SG_D_1_a7361), d_E_fd_SG_D_1_block/2(State_V_f_SG_D_1_1b8c0)
  psi_kq_SG_D_1/1 -> d_psi_q_SG_D_1_block/2(State_psi_kq_SG_D_1_b8294), d_psi_gq_SG_D_1_block/3(State_psi_kq_SG_D_1_82a75), d_psi_gq_SG_D_1_block/5(State_psi_kq_SG_D_1_01ca4), d_psi_kq_SG_D_1_block/4(State_psi_kq_SG_D_1_1418e), d_psi_kq_SG_D_1_block/2(State_psi_kq_SG_D_1_411eb), d_w_SG_D_1_block/5(State_psi_kq_SG_D_1_77cdd), d_psi_gq_SG_D_1_block/8(State_psi_kq_SG_D_1_4b627), d_V_f_SG_D_1_block/10(State_psi_kq_SG_D_1_518e4), i_d_SG_D_1_block/2(State_psi_kq_SG_D_1_f4c63), i_q_SG_D_1_block/2(State_psi_kq_SG_D_1_e7e60), T_e_SG_D_1_block/3(State_psi_kq_SG_D_1_d6793)
  w_SG_D_1_out_block/1(Blockout_w_SG_D_1_out_685b6) -> w_SG_D_1_out/1
  d_theta_SG_D_1_block/1(Blockout_d_theta_SG_D_1_4230e) -> theta_SG_D_1/1
  d_Px_1_SG_D_1_block/1(Blockout_d_Px_1_SG_D_1_adb46) -> Px_1_SG_D_1/1
  w_SG_D_1/1 -> d_psi_d_SG_D_1_block/9(State_w_SG_D_1_cd758), d_V_f_SG_D_1_block/13(State_w_SG_D_1_bdd46), d_w_SG_D_1_block/1(State_w_SG_D_1_243cd), d_psi_q_SG_D_1_block/9(State_w_SG_D_1_bb027), d_T_m_SG_D_1_block/1(State_w_SG_D_1_c0f9f), d_V_f_SG_D_1_block/8(State_w_SG_D_1_5e017), d_Px_2_SG_D_1_block/4(State_w_SG_D_1_35db8), d_Px_1_SG_D_1_block/2(State_w_SG_D_1_79126), d_Px_3_SG_D_1_block/6(State_w_SG_D_1_9ce72), d_theta_SG_D_1_block/1(State_w_SG_D_1_1d023), w_SG_D_1_out_block/1(State_w_SG_D_1_9c2ee)
  d_Px_3_SG_D_1_block/1(Blockout_d_Px_3_SG_D_1_3f1ef) -> Px_3_SG_D_1/1
  d_Px_2_SG_D_1_block/1(Blockout_d_Px_2_SG_D_1_bf890) -> Px_2_SG_D_1/1
  d_T_m_SG_D_1_block/1(Blockout_d_T_m_SG_D_1_8754a) -> T_m_SG_D_1/1
  psi_gq_SG_D_1/1 -> d_psi_q_SG_D_1_block/1(State_psi_gq_SG_D_1_7fe2e), d_psi_gq_SG_D_1_block/1(State_psi_gq_SG_D_1_82f3e), d_psi_gq_SG_D_1_block/2(State_psi_gq_SG_D_1_9fbdf), d_psi_gq_SG_D_1_block/4(State_psi_gq_SG_D_1_9b5fc), d_psi_kq_SG_D_1_block/1(State_psi_gq_SG_D_1_da5e1), d_psi_gq_SG_D_1_block/7(State_psi_gq_SG_D_1_9f3f0), i_q_SG_D_1_block/1(State_psi_gq_SG_D_1_7cf70), i_d_SG_D_1_block/1(State_psi_gq_SG_D_1_b21d8), d_V_f_SG_D_1_block/9(State_psi_gq_SG_D_1_ca757), d_w_SG_D_1_block/4(State_psi_gq_SG_D_1_917d5), d_psi_kq_SG_D_1_block/3(State_psi_gq_SG_D_1_e86a4), T_e_SG_D_1_block/2(State_psi_gq_SG_D_1_018b7)
  psi_fd_SG_D_1/1 -> d_psi_fd_SG_D_1_block/2(State_psi_fd_SG_D_1_493e7), d_psi_fd_SG_D_1_block/4(State_psi_fd_SG_D_1_c13e3), d_psi_fd_SG_D_1_block/7(State_psi_fd_SG_D_1_01812), d_psi_fd_SG_D_1_block/10(State_psi_fd_SG_D_1_d09aa), d_psi_d_SG_D_1_block/3(State_psi_fd_SG_D_1_4a659), d_psi_1d_SG_D_1_block/2(State_psi_fd_SG_D_1_06edd), d_w_SG_D_1_block/10(State_psi_fd_SG_D_1_4b2ae), d_V_f_SG_D_1_block/6(State_psi_fd_SG_D_1_66dec), i_d_SG_D_1_block/7(State_psi_fd_SG_D_1_12327), d_psi_1d_SG_D_1_block/5(State_psi_fd_SG_D_1_43462), i_q_SG_D_1_block/7(State_psi_fd_SG_D_1_87650), T_e_SG_D_1_block/8(State_psi_fd_SG_D_1_fa2b7)
  theta_SG_D_1/1 -> d_psi_d_SG_D_1_block/5(State_theta_SG_D_1_684aa), d_psi_q_SG_D_1_block/7(State_theta_SG_D_1_a61ef), i_d_SG_D_1_block/8(State_theta_SG_D_1_01785), d_psi_d_SG_D_1_block/7(State_theta_SG_D_1_1ab10), i_q_SG_D_1_block/8(State_theta_SG_D_1_ba088), i_d_SG_D_1_block/4(State_theta_SG_D_1_5398a), theta_SG_D_1_out_block/1(State_theta_SG_D_1_6aa7c), i_q_SG_D_1_block/4(State_theta_SG_D_1_65208), d_psi_q_SG_D_1_block/5(State_theta_SG_D_1_06da5)
  Px_1_SG_D_1/1 -> d_Px_2_SG_D_1_block/3(State_Px_1_SG_D_1_808d2), d_Px_3_SG_D_1_block/4(State_Px_1_SG_D_1_02f94), d_Px_3_SG_D_1_block/5(State_Px_1_SG_D_1_0957c), d_Px_2_SG_D_1_block/2(State_Px_1_SG_D_1_84ac5), d_Px_1_SG_D_1_block/1(State_Px_1_SG_D_1_40f75)
  v_d_SG_D_1/1 -> d_psi_d_SG_D_1_block/4(Input_v_d_SG_D_1_7e265), d_psi_q_SG_D_1_block/4(Input_v_d_SG_D_1_59a52)
  v_q_SG_D_1/1 -> d_psi_d_SG_D_1_block/6(Input_v_q_SG_D_1_b5510), d_psi_q_SG_D_1_block/6(Input_v_q_SG_D_1_df1d2)
  psi_q_SG_D_1/1 -> d_psi_d_SG_D_1_block/8(State_psi_q_SG_D_1_546c2), d_psi_q_SG_D_1_block/3(State_psi_q_SG_D_1_982cf), d_psi_gq_SG_D_1_block/6(State_psi_q_SG_D_1_bdf23), d_psi_gq_SG_D_1_block/9(State_psi_q_SG_D_1_96293), d_psi_kq_SG_D_1_block/5(State_psi_q_SG_D_1_82c28), d_w_SG_D_1_block/6(State_psi_q_SG_D_1_ca8e3), d_V_f_SG_D_1_block/7(State_psi_q_SG_D_1_48f64), d_w_SG_D_1_block/7(State_psi_q_SG_D_1_a45eb), d_V_f_SG_D_1_block/11(State_psi_q_SG_D_1_39754), i_d_SG_D_1_block/3(State_psi_q_SG_D_1_4cfdc), i_q_SG_D_1_block/3(State_psi_q_SG_D_1_51331), T_e_SG_D_1_block/4(State_psi_q_SG_D_1_b7612), T_e_SG_D_1_block/5(State_psi_q_SG_D_1_8370d)
  d_E_fd_SG_D_1_block/1(Blockout_d_E_fd_SG_D_1_9b618) -> E_fd_SG_D_1/1
  psi_1d_SG_D_1/1 -> d_psi_fd_SG_D_1_block/8(State_psi_1d_SG_D_1_43202), d_psi_fd_SG_D_1_block/5(State_psi_1d_SG_D_1_36641), d_psi_fd_SG_D_1_block/3(State_psi_1d_SG_D_1_737bf), d_psi_d_SG_D_1_block/1(State_psi_1d_SG_D_1_0a3f1), d_psi_1d_SG_D_1_block/1(State_psi_1d_SG_D_1_47359), d_psi_1d_SG_D_1_block/3(State_psi_1d_SG_D_1_6c7ce), d_w_SG_D_1_block/8(State_psi_1d_SG_D_1_85f69), d_V_f_SG_D_1_block/4(State_psi_1d_SG_D_1_b675d), i_d_SG_D_1_block/5(State_psi_1d_SG_D_1_b5c8c), T_e_SG_D_1_block/6(State_psi_1d_SG_D_1_c4246), i_q_SG_D_1_block/5(State_psi_1d_SG_D_1_b3786)
  Px_2_SG_D_1/1 -> d_Px_2_SG_D_1_block/1(State_Px_2_SG_D_1_536b3), d_Px_3_SG_D_1_block/2(State_Px_2_SG_D_1_ec984), d_Px_3_SG_D_1_block/3(State_Px_2_SG_D_1_b129a)
  psi_d_SG_D_1/1 -> d_psi_fd_SG_D_1_block/6(State_psi_d_SG_D_1_aa5d8), d_psi_fd_SG_D_1_block/9(State_psi_d_SG_D_1_d3017), d_psi_d_SG_D_1_block/2(State_psi_d_SG_D_1_d3b6a), d_psi_q_SG_D_1_block/8(State_psi_d_SG_D_1_9d031), d_psi_1d_SG_D_1_block/4(State_psi_d_SG_D_1_372e8), d_V_f_SG_D_1_block/5(State_psi_d_SG_D_1_9f482), i_q_SG_D_1_block/6(State_psi_d_SG_D_1_80107), T_e_SG_D_1_block/1(State_psi_d_SG_D_1_721af), i_d_SG_D_1_block/6(State_psi_d_SG_D_1_e1c0f), d_w_SG_D_1_block/3(State_psi_d_SG_D_1_7ac62), T_e_SG_D_1_block/7(State_psi_d_SG_D_1_20494), d_V_f_SG_D_1_block/12(State_psi_d_SG_D_1_d8f4d), d_w_SG_D_1_block/9(State_psi_d_SG_D_1_2f940)
  T_m_SG_D_1/1 -> d_T_m_SG_D_1_block/2(State_T_m_SG_D_1_2bf30), d_w_SG_D_1_block/2(State_T_m_SG_D_1_eee71)
  d_R_f_SG_D_1_block/1(Blockout_d_R_f_SG_D_1_f74b6) -> R_f_SG_D_1/1
  theta_SG_D_1_out_block/1(Blockout_theta_SG_D_1_out_3488a) -> theta_SG_D_1_out/1
  i_d_SG_D_1_block/1(Blockout_i_d_SG_D_1_dfa0a) -> i_d_SG_D_1/1
  i_q_SG_D_1_block/1(Blockout_i_q_SG_D_1_34308) -> i_q_SG_D_1/1
  T_e_SG_D_1_block/1(Blockout_T_e_SG_D_1_b08e1) -> T_e_SG_D_1/1
  d_psi_kq_SG_D_1_block/1(Blockout_d_psi_kq_SG_D_1_0e106) -> psi_kq_SG_D_1/1
  d_V_f_SG_D_1_block/1(Blockout_d_V_f_SG_D_1_17adf) -> V_f_SG_D_1/1
  d_psi_1d_SG_D_1_block/1(Blockout_d_psi_1d_SG_D_1_a3e0f) -> psi_1d_SG_D_1/1
  d_psi_q_SG_D_1_block/1(Blockout_d_psi_q_SG_D_1_a9dc6) -> psi_q_SG_D_1/1
  d_psi_gq_SG_D_1_block/1(Blockout_d_psi_gq_SG_D_1_8326c) -> psi_gq_SG_D_1/1
  d_psi_d_SG_D_1_block/1(Blockout_d_psi_d_SG_D_1_08662) -> psi_d_SG_D_1/1
  d_w_SG_D_1_block/1(Blockout_d_w_SG_D_1_52550) -> w_SG_D_1/1
  R_f_SG_D_1/1 -> d_V_f_SG_D_1_block/2(State_R_f_SG_D_1_58cf7), d_R_f_SG_D_1_block/2(State_R_f_SG_D_1_4464e)
  Px_3_SG_D_1/1 -> d_Px_3_SG_D_1_block/1(State_Px_3_SG_D_1_97912), d_V_f_SG_D_1_block/3(State_Px_3_SG_D_1_69e09)
  E_fd_SG_D_1/1 -> d_R_f_SG_D_1_block/1(State_E_fd_SG_D_1_91fb8), d_V_f_SG_D_1_block/1(State_E_fd_SG_D_1_2c396), d_E_fd_SG_D_1_block/1(State_E_fd_SG_D_1_e2b7b), d_psi_fd_SG_D_1_block/1(State_E_fd_SG_D_1_49e1f)
  d_psi_fd_SG_D_1_block/1(Blockout_d_psi_fd_SG_D_1_ef074) -> psi_fd_SG_D_1/1
